simulink model "Package_Baseline_Trajectory_Model"  (R2024a)
settings: Solver=VariableStepAuto  StartTime=0.0  StopTime=20.0  RelTol=1e-3
undefined symbols (not defined in the file): g, K_omega, K_p, k_r, K_v, Lambda, nu_b_0, Omega_r_0, p_b_i_0, q_0, R_turn_H, R_turn_V, T_max, T_min, UAV
libraries: matrix_library x1
settings Model: Creator=Usuario  LastModifiedBy=Usuario

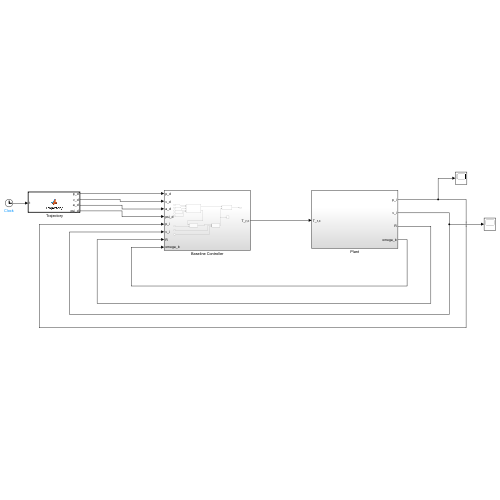
[thumbnail: Simulink's stored preview of the top-level diagram]
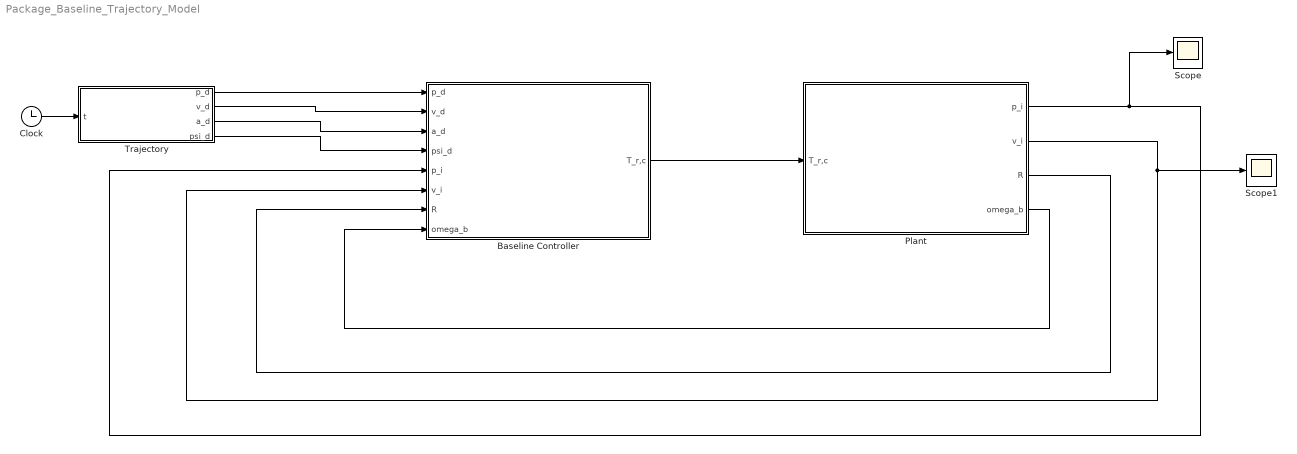
== system Package_Baseline_Trajectory_Model ==
  " Trajectory" : MATLAB Function  TreatAsAtomicUnit=on
  Baseline Controller : Subsystem
  Clock : Clock
  Plant : Subsystem
  Scope : Scope
  Scope1 : Scope
  wires:
  Clock/1 -> " Trajectory"/1(t)
  Baseline Controller/1(T_r,c) -> Plant/1(T_r,c)
  " Trajectory"/1(p_d) -> Baseline Controller/1(p_d)
  " Trajectory"/2(v_d) -> Baseline Controller/2(v_d)
  " Trajectory"/3(a_d) -> Baseline Controller/3(a_d)
  " Trajectory"/4(psi_d) -> Baseline Controller/4(psi_d)
  Plant/1(p_i) -> Scope/1, Baseline Controller/5(p_i)
  Plant/2(v_i) -> Baseline Controller/6(v_i), Scope1/1
  Plant/3(R) -> Baseline Controller/7(R)
  Plant/4(omega_b) -> Baseline Controller/8(omega_b)

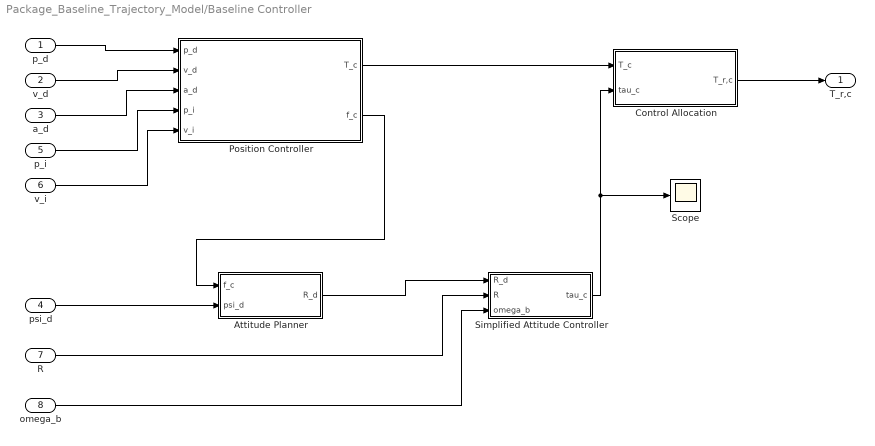
== system Package_Baseline_Trajectory_Model/Baseline Controller ==
  p_d : Inport
  v_d : Inport  Port=2
  a_d : Inport  Port=3
  psi_d : Inport  Port=4
  p_i : Inport  Port=5
  v_i : Inport  Port=6
  R : Inport  Port=7
  omega_b : Inport  Port=8
  Attitude Planner : Subsystem
  Control Allocation : Subsystem
  Position Controller : Subsystem
  Scope : Scope
  Simplified Attitude Controller : Subsystem
  T_r,c : Outport
  wires:
  Control Allocation/1(T_r,c) -> T_r,c/1
  p_d/1 -> Position Controller/1(p_d)
  v_d/1 -> Position Controller/2(v_d)
  a_d/1 -> Position Controller/3(a_d)
  Position Controller/1(T_c) -> Control Allocation/1(T_c)
  psi_d/1 -> Attitude Planner/2(psi_d)
  Position Controller/2(f_c) -> Attitude Planner/1(f_c)
  Attitude Planner/1(R_d) -> Simplified Attitude Controller/1(R_d)
  Simplified Attitude Controller/1(tau_c) -> Scope/1, Control Allocation/2(tau_c)
  p_i/1 -> Position Controller/4(p_i)
  v_i/1 -> Position Controller/5(v_i)
  R/1 -> Simplified Attitude Controller/2(R)
  omega_b/1 -> Simplified Attitude Controller/3(omega_b)

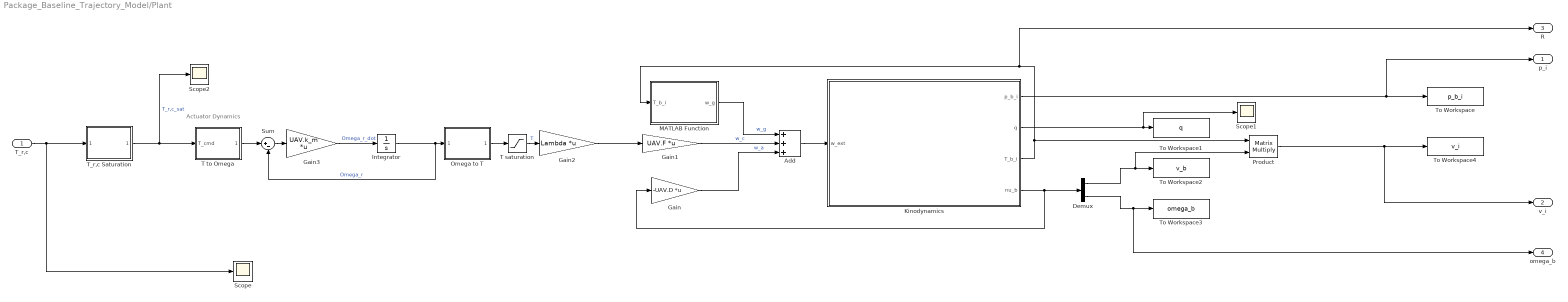
== system Package_Baseline_Trajectory_Model/Plant ==
  note: Actuator Dynamics
  T_r,c : Inport
  " Omega to T" : MATLAB Function  TreatAsAtomicUnit=on
  " T to Omega" : MATLAB Function  TreatAsAtomicUnit=on
  Add : Sum  Inputs=+++
  Demux : Demux  Outputs=[3 3]
  Gain : Gain  Gain=-UAV.D  Multiplication=Matrix(K*u)
  Gain1 : Gain  Gain=UAV.F  Multiplication=Matrix(K*u)
  Gain2 : Gain  Gain=Lambda  Multiplication=Matrix(K*u)
  Gain3 : Gain  Gain=UAV.k_m  Multiplication=Matrix(K*u)
  Integrator : Integrator  InitialCondition=Omega_r_0
  Kinodynamics : Subsystem
  MATLAB Function : MATLAB Function  TreatAsAtomicUnit=on
  Product : Product  Multiplication=Matrix(*)
  Scope : Scope
  Scope1 : Scope
  Scope2 : Scope
  Sum : Sum  Inputs=|+-
  T saturation : Saturate  UpperLimit=T_max  LowerLimit=T_min
  T_r,c Saturation : MATLAB Function  TreatAsAtomicUnit=on
  To Workspace : ToWorkspace  VariableName=p_b_i  SaveFormat=Timeseries  SampleTime=-1
  To Workspace1 : ToWorkspace  VariableName=q  SaveFormat=Timeseries  SampleTime=-1
  To Workspace2 : ToWorkspace  VariableName=v_b  SaveFormat=Timeseries  SampleTime=-1
  To Workspace3 : ToWorkspace  VariableName=omega_b  SaveFormat=Timeseries  SampleTime=-1
  To Workspace4 : ToWorkspace  VariableName=v_i  SaveFormat=Timeseries  SampleTime=-1
  p_i : Outport
  v_i : Outport  Port=2
  R : Outport  Port=3
  omega_b : Outport  Port=4
  wires:
  " T to Omega"/1(Omega_r_cmd) -> Sum/1
  Kinodynamics/3(T_b_i) -> R/1, MATLAB Function/1(T_b_i), Product/1
  Demux/2 -> omega_b/1, To Workspace3/1
  Kinodynamics/1(p_b_i) -> p_i/1, To Workspace/1
  Add/1 -> Kinodynamics/1(w_ext)
  Kinodynamics/4(nu_b) -> Gain/1, Demux/1
  Kinodynamics/2(q) -> Scope1/1, To Workspace1/1
  Product/1 -> v_i/1, To Workspace4/1
  Sum/1 -> Gain3/1
  Demux/1 -> Product/2, To Workspace2/1
  Gain/1 -> Add/3  "w_a"
  Gain1/1 -> Add/2  "w_c"
  Integrator/1 -> " Omega to T"/1(Omega_r), Sum/2  "Omega_r"
  MATLAB Function/1(w_g) -> Add/1  "w_g"
  Gain3/1 -> Integrator/1  "Omega_r_dot"
  T_r,c/1 -> T_r,c Saturation/1(Tr_cmd), Scope/1
  T_r,c Saturation/1(Tr_cmd_sat) -> Scope2/1, " T to Omega"/1(T_cmd)  "T_r,c_sat"
  " Omega to T"/1(T_ideal) -> T saturation/1
  T saturation/1 -> Gain2/1  "T"
  Gain2/1 -> Gain1/1

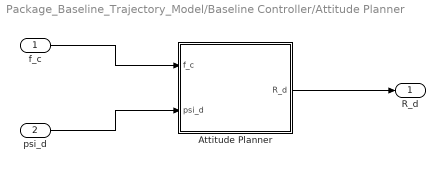
== system Package_Baseline_Trajectory_Model/Baseline Controller/Attitude Planner ==
  f_c : Inport
  psi_d : Inport  Port=2
  " Attitude Planner" : MATLAB Function  TreatAsAtomicUnit=on
  R_d : Outport
  wires:
  f_c/1 -> " Attitude Planner"/1(f_c)
  psi_d/1 -> " Attitude Planner"/2(psi_d)
  " Attitude Planner"/1(R_d) -> R_d/1

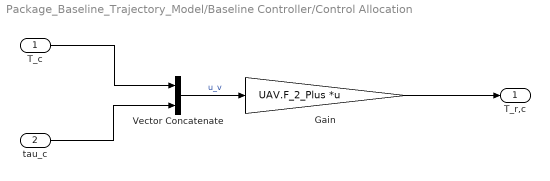
== system Package_Baseline_Trajectory_Model/Baseline Controller/Control Allocation ==
  T_c : Inport
  tau_c : Inport  Port=2
  Gain : Gain  Gain=UAV.F_2_Plus  Multiplication=Matrix(K*u)
  Vector Concatenate : Concatenate
  T_r,c : Outport
  wires:
  T_c/1 -> Vector Concatenate/1
  tau_c/1 -> Vector Concatenate/2
  Vector Concatenate/1 -> Gain/1  "u_v"
  Gain/1 -> T_r,c/1

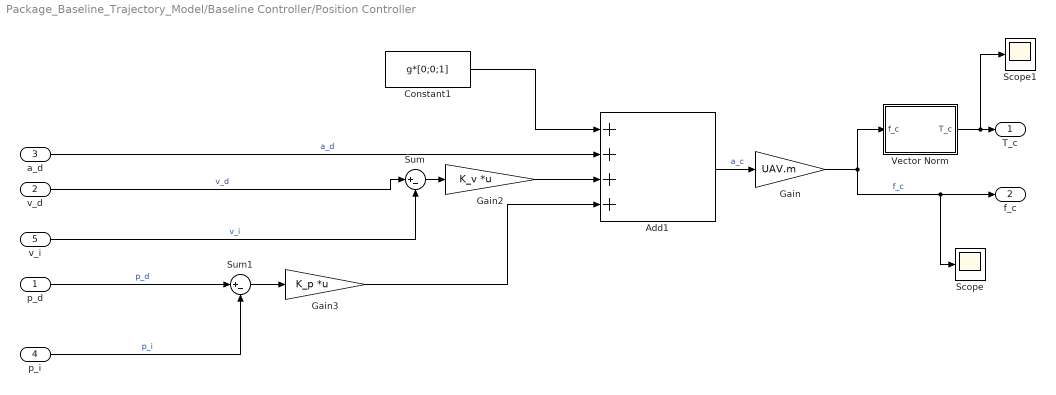
== system Package_Baseline_Trajectory_Model/Baseline Controller/Position Controller ==
  p_d : Inport
  v_d : Inport  Port=2
  a_d : Inport  Port=3
  p_i : Inport  Port=4
  v_i : Inport  Port=5
  Add1 : Sum  Inputs=++++
  Constant1 : Constant  Value=g*[0;0;1]
  Gain : Gain  Gain=UAV.m
  Gain2 : Gain  Gain=K_v  Multiplication=Matrix(K*u)
  Gain3 : Gain  Gain=K_p  Multiplication=Matrix(K*u)
  Scope : Scope
  Scope1 : Scope
  Sum : Sum  Inputs=|+-
  Sum1 : Sum  Inputs=|+-
  Vector Norm : MATLAB Function  TreatAsAtomicUnit=on
  T_c : Outport
  f_c : Outport  Port=2
  wires:
  p_d/1 -> Sum1/1  "p_d"
  Gain3/1 -> Add1/4
  Sum1/1 -> Gain3/1
  Sum/1 -> Gain2/1
  Gain2/1 -> Add1/3
  a_d/1 -> Add1/2  "a_d"
  Constant1/1 -> Add1/1
  v_d/1 -> Sum/1  "v_d"
  Add1/1 -> Gain/1  "a_c"
  p_i/1 -> Sum1/2  "p_i"
  v_i/1 -> Sum/2  "v_i"
  Gain/1 -> Vector Norm/1(f_c), Scope/1, f_c/1  "f_c"
  Vector Norm/1(T_c) -> Scope1/1, T_c/1

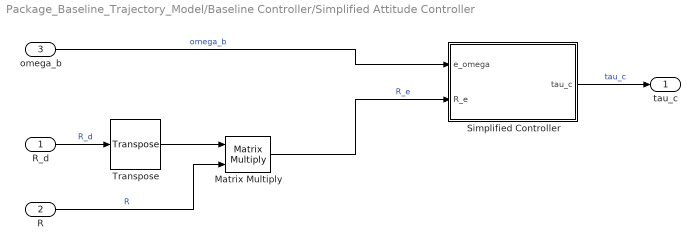
== system Package_Baseline_Trajectory_Model/Baseline Controller/Simplified Attitude Controller ==
  R_d : Inport
  R : Inport  Port=2
  omega_b : Inport  Port=3
  Matrix Multiply : Product  Multiplication=Matrix(*)
  Simplified Controller : MATLAB Function  TreatAsAtomicUnit=on
  Transpose : matrix_library/Transpose
  tau_c : Outport
  wires:
  omega_b/1 -> Simplified Controller/1(e_omega)  "omega_b"
  Matrix Multiply/1 -> Simplified Controller/2(R_e)  "R_e"
  Transpose/1 -> Matrix Multiply/1
  R_d/1 -> Transpose/1  "R_d"
  Simplified Controller/1(tau_c) -> tau_c/1  "tau_c"
  R/1 -> Matrix Multiply/2  "R"

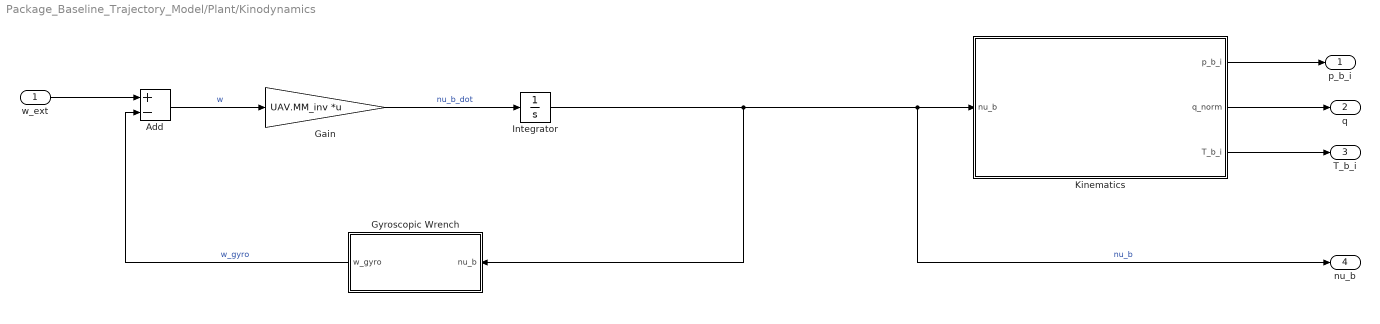
== system Package_Baseline_Trajectory_Model/Plant/Kinodynamics ==
  w_ext : Inport
  Add : Sum  Inputs=+-
  Gain : Gain  Gain=UAV.MM_inv  Multiplication=Matrix(K*u)
  Gyroscopic Wrench : MATLAB Function  TreatAsAtomicUnit=on
  Integrator : Integrator  InitialCondition=nu_b_0
  Kinematics : Subsystem
  p_b_i : Outport
  q : Outport  Port=2
  T_b_i : Outport  Port=3
  nu_b : Outport  Port=4
  wires:
  Kinematics/1(p_b_i) -> p_b_i/1
  w_ext/1 -> Add/1
  Integrator/1 -> Gyroscopic Wrench/1(nu_b), nu_b/1, Kinematics/1(nu_b)  "nu_b"
  Gain/1 -> Integrator/1  "nu_b_dot"
  Kinematics/3(T_b_i) -> T_b_i/1
  Kinematics/2(q_norm) -> q/1
  Gyroscopic Wrench/1(w_gyro) -> Add/2  "w_gyro"
  Add/1 -> Gain/1  "w"

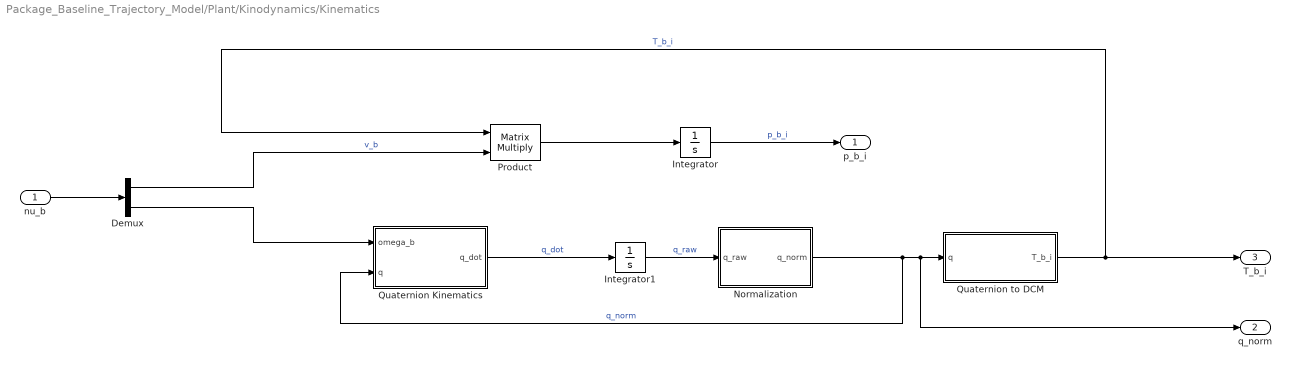
== system Package_Baseline_Trajectory_Model/Plant/Kinodynamics/Kinematics ==
  nu_b : Inport
  " Normalization" : MATLAB Function  TreatAsAtomicUnit=on
  Demux : Demux  Outputs=[3 3]
  Integrator : Integrator  InitialCondition=p_b_i_0
  Integrator1 : Integrator  InitialCondition=q_0
  Product : Product  Multiplication=Matrix(*)
  Quaternion Kinematics : MATLAB Function  TreatAsAtomicUnit=on
  Quaternion to DCM : MATLAB Function  TreatAsAtomicUnit=on
  p_b_i : Outport
  q_norm : Outport  Port=2
  T_b_i : Outport  Port=3
  wires:
  Integrator1/1 -> " Normalization"/1(q_raw)  "q_raw"
  " Normalization"/1(q_norm) -> Quaternion to DCM/1(q), q_norm/1, Quaternion Kinematics/2(q)  "q_norm"
  Demux/2 -> Quaternion Kinematics/1(omega_b)
  Quaternion Kinematics/1(q_dot) -> Integrator1/1  "q_dot"
  Product/1 -> Integrator/1
  Quaternion to DCM/1(T_b_i) -> T_b_i/1, Product/1  "T_b_i"
  Demux/1 -> Product/2  "v_b"
  Integrator/1 -> p_b_i/1  "p_b_i"
  nu_b/1 -> Demux/1

== matlab function Package_Baseline_Trajectory_Model/Baseline Controller/Simplified Attitude Controller/Simplified Controller ==
  data: e_omega input; tau_c output; R_e input; k_r parameter; K_omega parameter
function tau_c=Controller(e_omega,R_e,k_r, K_omega)
%Construct er
e_r=zeros(3,1);
I=eye(3,3);
for i=1:3
    e_r=e_r+k_r(i)*cross_matrix(R_e'*I(:,i))*I(:,i);
end
%Construct tau_c
tau_c=-e_r-K_omega*e_omega;

end

== matlab function Package_Baseline_Trajectory_Model/Plant/Kinodynamics/Kinematics/Quaternion to DCM ==
  data: q input; T_b_i output
function T_b_i=quaternion_to_DCM(q)
%My implementation of the quaternion to DCM transformation, to ensure
%consistency. It must return the active representation of the rotation
%between i and b, which will be the DCM from b to i. 
eta=q(1);
epsilon=q(2:4);
epsilon_x=cross_matrix(epsilon);

T_b_i=eye(3,3)+2*eta*epsilon_x+2*epsilon_x*epsilon_x;
end

== matlab function Package_Baseline_Trajectory_Model/Plant/Kinodynamics/Kinematics/ Normalization ==
  data: q_raw input; q_norm output
function q_norm=normalization(q_raw)

q_norm=q_raw/norm(q_raw);

== matlab function Package_Baseline_Trajectory_Model/Plant/Kinodynamics/Kinematics/Quaternion Kinematics ==
  data: omega_b input; q_dot output; q input
function q_dot = quat_kinematics(omega_b,q)
%Quaternion kinematics. Requires that omega_b be a column vector. q must
%also be a column vector following the course's quaternion convention. 
eta=q(1);
epsilon=q(2:4);
epsilon_x=cross_matrix(epsilon);

q_dot=1/2*[-epsilon';epsilon_x+eta*eye(3,3)]*omega_b;
end

== matlab function Package_Baseline_Trajectory_Model/Plant/Kinodynamics/Gyroscopic Wrench ==
  data: nu_b input; w_gyro output; UAV parameter
function w_gyro=gyroscopic_wrench(nu_b,UAV)
nu_b_southwest=[cross_matrix(nu_b(4:6)),zeros(3,3);cross_matrix(nu_b(1:3)),cross_matrix(nu_b(4:6))];
w_gyro=nu_b_southwest*UAV.MM*nu_b;
end

== matlab function Package_Baseline_Trajectory_Model/Plant/MATLAB Function ==
  data: T_b_i input; w_g output; UAV parameter; g parameter
function w_g=Gravity_Wrench(T_b_i,UAV, g)
e3=[0;0;1];

w_g=-g*[UAV.m*T_b_i'*e3;UAV.S_t*T_b_i'*e3];
end

== matlab function Package_Baseline_Trajectory_Model/Plant/ T to Omega ==
  data: T_cmd input; Omega_r_cmd output; k_f parameter
function Omega_r_cmd=T_to_Omega(T_cmd,k_f)
Omega_r_cmd=sqrt(T_cmd/k_f);
end

== matlab function Package_Baseline_Trajectory_Model/Plant/ Omega to T ==
  data: Omega_r input; T_ideal output; k_f parameter
function T_ideal=Omega_to_T(Omega_r,k_f)
T_ideal=k_f*Omega_r.^2;
end

== matlab function Package_Baseline_Trajectory_Model/ Trajectory ==
  data: t input; p_d output; v_d output; a_d output; psi_d output; R_turn_V parameter; R_turn_H parameter
function [p_d,v_d,a_d,psi_d]=Trajectory(t,R_turn_V,R_turn_H)
%This function must take in time and return the desired position, velocity,
%acceleration and heading angle of the trajectory one wants the UAV to
%track. For now, I will leave it as a placeholder. 
[p_d,v_d,a_d,psi_d]=representative_trajectory(t,R_turn_V,R_turn_H);
end

== matlab function Package_Baseline_Trajectory_Model/Baseline Controller/Position Controller/Vector Norm ==
  data: f_c input; T_c output
function T_c=norm(f_c)
T_c=norm(f_c);
end

== matlab function Package_Baseline_Trajectory_Model/Baseline Controller/Attitude Planner/ Attitude Planner ==
  data: f_c input; R_d output; psi_d input
function R_d=Attitude_Planner(f_c,psi_d)
%This function implements the attitude planner logic in P2CS1. It
%constructs the expression of the basis vectors of the desired attitude in 
%the inertial frame and uses them to construct R_d. For details, see slides.  
k_p_i=f_c/norm(f_c);
h_d_i=[cos(psi_d);sin(psi_d);0];
j_p_i=cross(k_p_i,h_d_i)/norm(cross(k_p_i,h_d_i));
i_p_i=cross(j_p_i,k_p_i)/norm(cross(j_p_i,k_p_i)); %normalization not necessary in theory, but I implement it just in case there are some numerical errors.

R_d=[i_p_i,j_p_i,k_p_i];
end

== matlab function Package_Baseline_Trajectory_Model/Plant/T_r,c Saturation ==
  data: Tr_cmd input; Tr_cmd_sat output; T_min parameter; T_max parameter
function Tr_cmd_sat=Command_Input_Saturation(Tr_cmd,T_min, T_max)
Tr_cmd_sat=nan(size(Tr_cmd));
for i=1:length(Tr_cmd)
    if Tr_cmd(i)<T_min
        Tr_cmd_sat(i)=T_min;
    elseif Tr_cmd(i)>T_max
        Tr_cmd_sat(i)=T_max;
    else
        Tr_cmd_sat(i)=Tr_cmd(i);
    end
end
end
